simulink model "rotation_controllers_energy_test"  (Simulink 8.8)
settings: Solver=ode4  StartTime=0.0  StopTime=10.0  FixedStep=1e-4  RelTol=1e-3  EnableMultiTasking=on
values from neighbouring files (symbols this model uses):
  g_W = [0;0;-9.81]    [rotation_controllers_energy_test_start.m]
  I_B1_C1 = inertiavector2matrix([2, 3, 12,0,-3,-0.2])    [rotation_controllers_energy_test_start.m]
  I_B2_C2 = inertiavector2matrix([4, 8, 15,-1,-2,-0.5])    [rotation_controllers_energy_test_start.m]
  m1 = 1    [rotation_controllers_energy_test_start.m]
  m2 = 1.5    [rotation_controllers_energy_test_start.m]
  r_B1_C1_F1 = -r_B1_B1_C1+r_B1_B1_F1    [rotation_controllers_energy_test_start.m]
  r_B2_C2_F2 = -r_B2_B2_C2+r_B2_B2_F2    [rotation_controllers_energy_test_start.m]
undefined symbols (not defined in the file): k_D_p, k_D_r, k_P_p, k_P_r
libraries: lib_rigid_body_kinematics x8, lib_rigid_body_dynamics x6, lib_transformations x4, lib_cartesian_controllers x2, vrlib x2
settings Model: SuppressorTable=22 serialization::archive 11 0 3 0 0 0 11 0  Creator=schappler  LastModifiedBy=schappler
settings DataIOCC: LimitDataPoints=off  SaveFormat=StructureWithTime  SignalLoggingSaveFormat=Dataset
settings DebuggingCC: UnderspecifiedInitializationDetection=Simplified  MergeDetectMultiDrivingBlocksExec=error  FcnCallInpInsideContextMsg=error  StateNameClashWarn=none
settings GRTTargetCC: CombineOutputUpdateFcns=on  GRTInterface=off

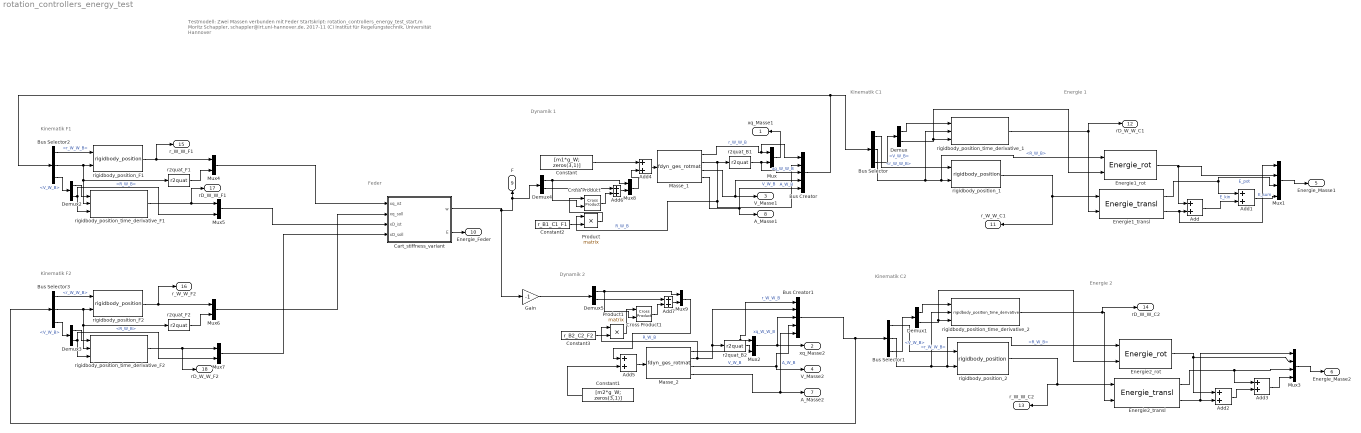
== system rotation_controllers_energy_test ==
  note: Testmodell: Zwei Massen verbunden mit Feder
      | Startskript: rotation_controllers_energy_test_start.m
      |
      | Moritz Schappler, schappler@irt.uni-hannover.de, 2017-11
      | (C) Institut für Regelungstechnik, Universität Hannover
  note: Kinematik C2
  note: Kinematik C1
  note: Dynamik 2
  note: Dynamik 1
  note: Feder
  note: Kinematik F1
  note: Energie 1
  note: Energie 2
  note: Kinematik F2
  Add{,1..7} (8 alike) : Sum
  Bus Creator : BusCreator  Inputs=5
  Bus Creator1 : BusCreator  Inputs=5
  Bus Selector{,1..3} (4 alike) : BusSelector  OutputSignals=r_W_W_B,R_W_B,V_W_B
  Cart_stiffness_variant : Subsystem  Variant=on  mask{K_P_p=k_P_p, k_P_r=k_P_r, k_D_p=k_D_p, k_D_r=k_D_r}
  Constant : Constant  Value=[m1*g_W; zeros(3,1)]
  Constant1 : Constant  Value=[m2*g_W; zeros(3,1)]
  Constant2 : Constant  Value=r_B1_C1_F1
  Constant3 : Constant  Value=r_B2_C2_F2
  Cross Product : vrlib/Utilities/Cross Product
  Cross Product1 : vrlib/Utilities/Cross Product
  Demux{,1,4..5} (4 alike) : Demux  Outputs=2
  Demux2 : Demux  Outputs=[3 3]
  Demux3 : Demux  Outputs=[3 3]
  Energie1_rot : lib_rigid_body_dynamics/Energie_rot  I_B_C=I_B1_C1
  Energie1_transl : lib_rigid_body_dynamics/Energie_transl  m=m1  g_W=g_W
  Energie2_rot : lib_rigid_body_dynamics/Energie_rot  I_B_C=I_B2_C2
  Energie2_transl : lib_rigid_body_dynamics/Energie_transl  m=m2  g_W=g_W
  Gain : Gain  Gain=-1
  Masse_1 : lib_rigid_body_dynamics/fdyn_ges_rotmat  I=I_B1_C1  m=m1  r0=r_W_W_B1_t0  rD0=rD_W_W_B1_t0  R_t0=R_W_B1_t0  omega0_t0=omega_W_B1_t0  r_B_B_C=r_B1_B1_C1
  Masse_2 : lib_rigid_body_dynamics/fdyn_ges_rotmat  I=I_B2_C2  m=m2  r0=r_W_W_B2_t0  rD0=rD_W_W_B2_t0  R_t0=R_W_B2_t0  omega0_t0=omega_W_B2_t0  r_B_B_C=r_B2_B2_C2
  Mux{,2,4,6} (4 alike) : Mux  Inputs=[3 4]
  Mux1 : Mux  Inputs=[1 1 1 1]
  Mux3 : Mux  Inputs=[1 1 1 1]
  Mux{5,7..9} (4 alike) : Mux  Inputs=[3 3]
  Product : Product  Multiplication=Matrix(*)
  Product1 : Product  Multiplication=Matrix(*)
  r2quat_B1 : lib_transformations/r2quat
  r2quat_B2 : lib_transformations/r2quat
  r2quat_F1 : lib_transformations/r2quat
  r2quat_F2 : lib_transformations/r2quat
  rigidbody_position_1 : lib_rigid_body_kinematics/rigidbody_position  r_B_B_C=r_B1_B1_C1  PktName_B='B1'  PktName_C='C1'  KSName_W='W'
  rigidbody_position_2 : lib_rigid_body_kinematics/rigidbody_position  r_B_B_C=r_B2_B2_C2  PktName_B='B2'  PktName_C='C2'  KSName_W='W'
  rigidbody_position_F1 : lib_rigid_body_kinematics/rigidbody_position  r_B_B_C=r_B1_B1_F1  PktName_B='B1'  PktName_C='F1'  KSName_W='W'
  rigidbody_position_F2 : lib_rigid_body_kinematics/rigidbody_position  r_B_B_C=r_B2_B2_F2  PktName_B='B2'  PktName_C='F2'  KSName_W='W'
  rigidbody_position_time_derivative_1 : lib_rigid_body_kinematics/rigidbody_position_time_derivative  r_B_B_C=r_B1_B1_C1  PktName_B='B1'  PktName_C='C1'  KSName_W='W'
  rigidbody_position_time_derivative_2 : lib_rigid_body_kinematics/rigidbody_position_time_derivative  r_B_B_C=r_B2_B2_C2  PktName_B='B2'  PktName_C='C2'  KSName_W='W'
  rigidbody_position_time_derivative_F1 : lib_rigid_body_kinematics/rigidbody_position_time_derivative  r_B_B_C=r_B1_B1_F1  PktName_B='B1'  PktName_C='F1'  KSName_W='W'
  rigidbody_position_time_derivative_F2 : lib_rigid_body_kinematics/rigidbody_position_time_derivative  r_B_B_C=r_B2_B2_F2  PktName_B='B2'  PktName_C='F2'  KSName_W='W'
  xq_Masse1 : Outport
  xq_Masse2 : Outport  Port=2
  V_Masse1 : Outport  Port=3
  V_Masse2 : Outport  Port=4
  Energie_Masse1 : Outport  Port=5
  Energie_Masse2 : Outport  Port=6
  A_Masse2 : Outport  Port=7
  A_Masse1 : Outport  Port=8
  F : Outport  Port=9
  Energie_Feder : Outport  Port=10
  r_W_W_C1 : Outport  Port=11
  rD_W_W_C1 : Outport  Port=12
  r_W_W_C2 : Outport  Port=13
  rD_W_W_C2 : Outport  Port=14
  r_W_W_F1 : Outport  Port=15
  r_W_W_F2 : Outport  Port=16
  rD_W_W_F1 : Outport  Port=17
  rD_W_W_F2 : Outport  Port=18
  wires:
  Masse_1/2 -> Product/1, Bus Creator/2, r2quat_B1/1  "R_W_B"
  r2quat_B1/1 -> Bus Creator/3, Mux/2  "xq_W_W_B"
  Masse_1/1 -> Bus Creator/1, Mux/1  "r_W_W_B"
  Mux/1 -> xq_Masse1/1
  r2quat_B2/1 -> Mux2/2
  Mux2/1 -> Bus Creator1/3, xq_Masse2/1  "xq_W_W_B"
  Masse_1/3 -> Bus Creator/4, V_Masse1/1  "V_W_B"
  Demux/2 -> Energie1_rot/2, rigidbody_position_time_derivative_1/3
  Energie1_transl/2 -> Mux1/1, Add/2
  Add/1 -> Add1/2  "E_kin"
  Energie1_rot/1 -> Mux1/2, Add/1
  Energie1_transl/1 -> Mux1/3, Add1/1  "E_pot"
  Add1/1 -> Mux1/4  "E_sum"
  Mux1/1 -> Energie_Masse1/1
  rigidbody_position_1/1 -> r_W_W_C1/1, Energie1_transl/1
  Demux/1 -> rigidbody_position_time_derivative_1/1
  rigidbody_position_time_derivative_1/1 -> rD_W_W_C1/1, Energie1_transl/2
  Masse_2/2 -> Bus Creator1/2, r2quat_B2/1, Product1/1  "R_W_B"
  Masse_2/1 -> Bus Creator1/1, Mux2/1  "r_W_W_B"
  Masse_2/3 -> V_Masse2/1, Bus Creator1/4  "V_W_B"
  Demux1/2 -> Energie2_rot/2, rigidbody_position_time_derivative_2/3
  Energie2_transl/2 -> Mux3/1, Add2/2
  Add2/1 -> Add3/2
  Energie2_rot/1 -> Mux3/2, Add2/1
  Energie2_transl/1 -> Mux3/3, Add3/1
  Add3/1 -> Mux3/4
  Mux3/1 -> Energie_Masse2/1
  rigidbody_position_2/1 -> r_W_W_C2/1, Energie2_transl/1
  Demux1/1 -> rigidbody_position_time_derivative_2/1
  rigidbody_position_time_derivative_2/1 -> rD_W_W_C2/1, Energie2_transl/2
  Masse_2/4 -> Bus Creator1/5, A_Masse2/1  "A_W_B"
  Masse_1/4 -> Bus Creator/5, A_Masse1/1  "A_W_B"
  Constant/1 -> Add4/1
  Add5/1 -> Masse_2/1
  Add4/1 -> Masse_1/1
  Constant1/1 -> Add5/2
  Cart_stiffness_variant/2(E) -> Energie_Feder/1
  Cart_stiffness_variant/1(w) -> Gain/1, Demux4/1, F/1
  Bus Creator/1 -> Bus Selector2/1, Bus Selector/1
  Bus Selector/3 -> Demux/1  "<V_W_B>"
  Bus Selector/1 -> rigidbody_position_1/1  "<r_W_W_B>"
  Bus Selector/2 -> rigidbody_position_time_derivative_1/2, Energie1_rot/1, rigidbody_position_1/2  "<R_W_B>"
  Bus Creator1/1 -> Bus Selector3/1, Bus Selector1/1
  Bus Selector1/3 -> Demux1/1  "<V_W_B>"
  Bus Selector1/1 -> rigidbody_position_2/1  "<r_W_W_B>"
  Bus Selector1/2 -> rigidbody_position_time_derivative_2/2, Energie2_rot/1, rigidbody_position_2/2  "<R_W_B>"
  Bus Selector2/1 -> rigidbody_position_F1/1  "<r_W_W_B>"
  Bus Selector2/2 -> r2quat_F1/1, rigidbody_position_time_derivative_F1/2, rigidbody_position_F1/2  "<R_W_B>"
  Bus Selector2/3 -> Demux2/1  "<V_W_B>"
  Demux2/1 -> rigidbody_position_time_derivative_F1/1
  Demux2/2 -> rigidbody_position_time_derivative_F1/3, Mux5/2
  rigidbody_position_F1/1 -> r_W_W_F1/1, Mux4/1
  r2quat_F1/1 -> Mux4/2
  Mux4/1 -> Cart_stiffness_variant/1(xq_ist)
  rigidbody_position_time_derivative_F1/1 -> rD_W_W_F1/1, Mux5/1
  Mux5/1 -> Cart_stiffness_variant/3(xD_ist)
  Bus Selector3/1 -> rigidbody_position_F2/1  "<r_W_W_B>"
  Bus Selector3/2 -> r2quat_F2/1, rigidbody_position_time_derivative_F2/2, rigidbody_position_F2/2  "<R_W_B>"
  Bus Selector3/3 -> Demux3/1  "<V_W_B>"
  Demux3/1 -> rigidbody_position_time_derivative_F2/1
  Demux3/2 -> rigidbody_position_time_derivative_F2/3, Mux7/2
  rigidbody_position_F2/1 -> r_W_W_F2/1, Mux6/1
  r2quat_F2/1 -> Mux6/2
  Mux6/1 -> Cart_stiffness_variant/2(xq_soll)
  rigidbody_position_time_derivative_F2/1 -> rD_W_W_F2/1, Mux7/1
  Mux7/1 -> Cart_stiffness_variant/4(xD_soll)
  Demux4/1 -> Cross Product/2, Mux8/1
  Add6/1 -> Mux8/2
  Demux4/2 -> Add6/1
  Constant2/1 -> Product/2
  Product/1 -> Cross Product/1
  Cross Product/1 -> Add6/2
  Mux8/1 -> Add4/2
  Gain/1 -> Demux5/1
  Demux5/1 -> Cross Product1/2, Mux9/1
  Add7/1 -> Mux9/2
  Demux5/2 -> Add7/1
  Constant3/1 -> Product1/2
  Product1/1 -> Cross Product1/1
  Cross Product1/1 -> Add7/2
  Mux9/1 -> Add5/1

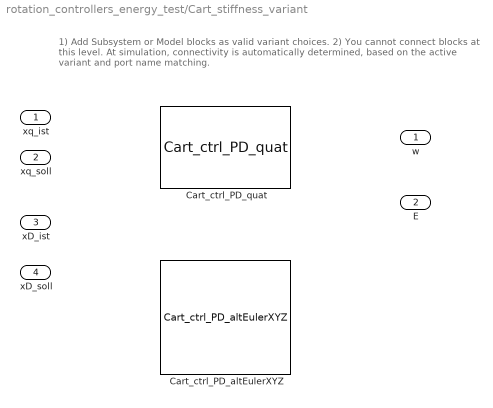
== system rotation_controllers_energy_test/Cart_stiffness_variant ==
  note: 1) Add Subsystem or Model blocks as valid variant choices.
      | 2) You cannot connect blocks at this level. At simulation, connectivity is automatically
      | determined, based on the active variant and port name matching.
  xq_ist : Inport
  xq_soll : Inport  Port=2
  xD_ist : Inport  Port=3
  xD_soll : Inport  Port=4
  Cart_ctrl_PD_altEulerXYZ : lib_cartesian_controllers/Cart_ctrl_PD_altEulerXYZ  VariantControl=CART_CONTROLLER_EULER  k_P_p=k_P_p  k_P_r=k_P_r  k_D_p=k_D_p  k_D_r=k_D_r
  Cart_ctrl_PD_quat : lib_cartesian_controllers/Cart_ctrl_PD_quat  VariantControl=CART_CONTROLLER_QUATERNION  k_P_p=k_P_p  k_P_r=k_P_r  k_D_p=k_D_p  k_D_r=k_D_r
  w : Outport
  E : Outport  Port=2
